simulink model "sf_varsize_example"  (R2017b)
settings: Solver=FixedStepDiscrete  StartTime=0.0  StopTime=inf  FixedStep=0.05  RelTol=1e-3  EnableMultiTasking=on
settings Model: Creator=The MathWorks, Inc.  LastModifiedBy=The MathWorks, Inc.
settings DataIOCC: LimitDataPoints=on  SaveFormat=Array
settings OptimizationCC: ExpressionDepthLimit=2147483647  LifeSpan=inf
settings DebuggingCC: UnderspecifiedInitializationDetection=Classic  MergeDetectMultiDrivingBlocksExec=none  SolverPrmCheckMsg=warning  FcnCallInpInsideContextMsg=warning  StateNameClashWarn=warning  StrictBusMsg=Warning  SFUnexpectedBacktrackingDiag=warning  SFNoUnconditionalDefaultTransitionDiag=warning  SFExecutionAtInitializationDiag=none
settings HardwareCC: ProdBitPerPointer=32  ProdBitPerSizeT=32  ProdBitPerPtrDiffT=32  ProdLargestAtomicFloat=None  ProdIntDivRoundTo=Undefined  ProdEndianess=Unspecified  ProdWordSize=32  ProdHWDeviceType=32-bit Generic
settings ModelReferenceCC: PropagateSignalLabelsOutOfModel=off
settings SFSimCC: SimParseCustomCode=off
settings CodeAppCC: StateflowObjectComments=on
settings GRTTargetCC: TargetLangStandard=C89/C90 (ANSI)  GeneratePreprocessorConditionals=Disable all  CombineOutputUpdateFcns=off  GRTInterface=on
settings ConfigComp: CovMetricSettings=dw  CovHtmlReporting=on  CovSaveCumulativeToWorkspaceVar=on  CovSaveSingleToWorkspaceVar=on  CovExternalEMLEnable=off  CovSFcnEnable=off

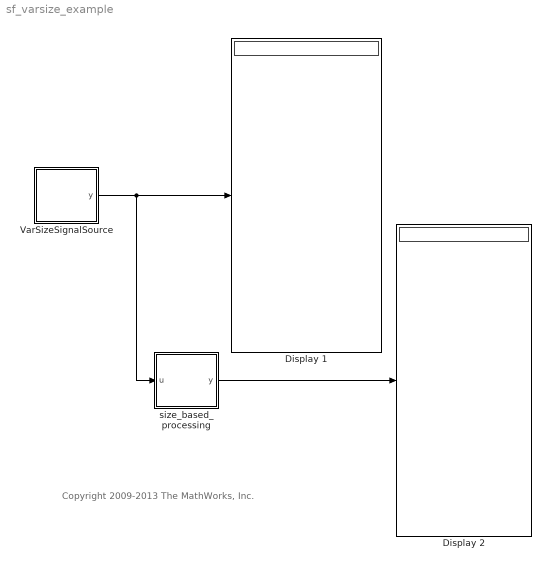
== system sf_varsize_example ==
  note: Copyright 2009-2013 The MathWorks, Inc.
  Display 1 : Display
  Display 2 : Display
  VarSizeSignalSource : Stateflow chart  TreatAsAtomicUnit=on
  size_based_processing : Stateflow chart  TreatAsAtomicUnit=on
  wires:
  VarSizeSignalSource/1(y) -> Display 1/1, size_based_processing/1(u)
  size_based_processing/1(y) -> Display 2/1

== stateflow chart sf_varsize_example/VarSizeSignalSource ==
  state Scalar
    en: generateOutput(1);
    du: generateOutput(1);
  state VectorFull
    en: generateOutput(16);
    du: generateOutput(16);
  state VectorPartial
    en: generateOutput(8);
    du: generateOutput(8);
  note: Use this Stateflow chart to generate an output signal with a variable size.  In this chart,
      | each state calls a MATLAB function that assigns to the chart output
      | a different-sized signal (within the bounds).  During simulation, transitions between states
      | change the size of the signal. You can use this variable-size signal to test other blocks
      | and subsystems in your model.
  (default) -> Scalar
  VectorFull -> Scalar : [after(5,tick)]
  Scalar -> VectorPartial : [after(5,tick)]
  VectorPartial -> VectorFull : [after(5,tick)]
  data: len function_input double; y output double size=16
  function generateOutput(len):
    | function generateOutput(len)
    | %#codegen
    | assert(len<=16);
    | y = (1:len)';

== stateflow chart sf_varsize_example/size_based_processing ==
  state Scalar
    entry: reset_output();
  state Vector
    en: compute_output();
    du: compute_output();
  note: In this chart, MATLAB functions:
      | (a) Determine the size of the input signal.
      | (b) Use MATLAB syntax to compute variable-size outputs based on inputs.
      | (c) Reset the output to zero when the input is scalar.
      |
      | Key behavior:
      | 1. Variable-size data are allowed only for chart input and output data.
      | 2. Variable-size data "u" and "y" do not appear in state actions or on transitions.
      | 3. MATLAB functions access variable-size data "u" and y" directly for computations.
      | 4. MATLAB functions do not use variable dimensions for their own input and output data.
  (default) -> Scalar
  Vector -> Scalar : [is_scalar_input()]
  Scalar -> Vector : [~is_scalar_input()]
  data: isScalar function_output boolean; u input double size=16; y output double size=16
  function reset_output:
    | function reset_output
    | %#codegen
    | y = 0;
  function compute_output:
    | function compute_output
    | %#codegen
    | y = sin(u);
  function isScalar = is_scalar_input:
    | function isScalar = is_scalar_input
    | %#codegen
    | isScalar = length(u)==1;
